simulink model "Task1_Simulink"  (R2023b)
settings: Solver=VariableStepAuto  StartTime=0.0  StopTime=10.0  RelTol=1e-3
values from neighbouring files (symbols this model uses):
  k = find(modeldata.studentList == studentNo)    [runExam.m]
undefined symbols (not defined in the file or in its folder): b, g, m, theta1, theta2, zk
settings Model: Creator=qnmdgpqs  LastModifiedBy=qnmdgpqs

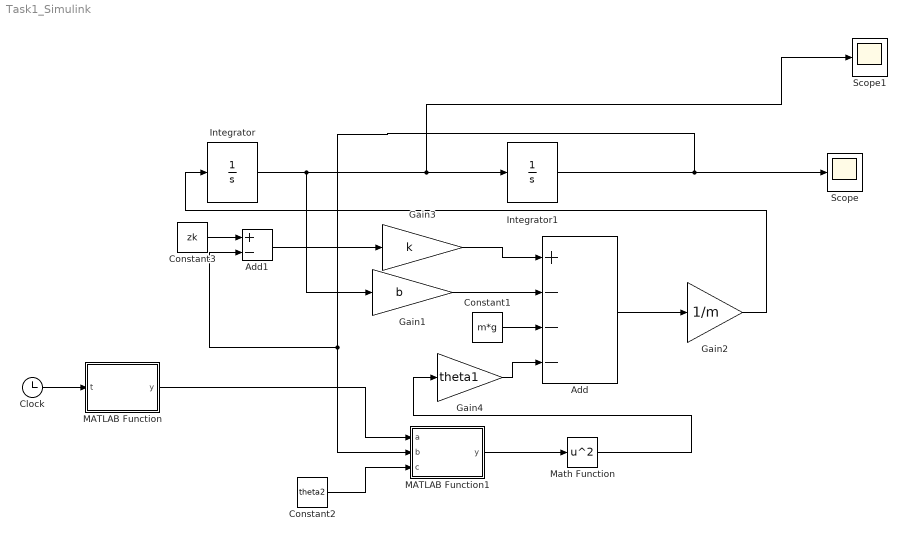
== system Task1_Simulink ==
  Add : Sum  Inputs=+---
  Add1 : Sum  Inputs=+-
  Clock : Clock
  Constant1 : Constant  Value=m*g
  Constant2 : Constant  Value=theta2
  Constant3 : Constant  Value=zk
  Gain1 : Gain  Gain=b
  Gain2 : Gain  Gain=1/m
  Gain3 : Gain  Gain=k
  Gain4 : Gain  Gain=theta1
  Integrator : Integrator
  Integrator1 : Integrator  InitialCondition=0.1
  MATLAB Function : MATLAB Function  TreatAsAtomicUnit=on
  MATLAB Function1 : MATLAB Function  TreatAsAtomicUnit=on
  Math Function : Math  Operator=square
  Scope : Scope
  Scope1 : Scope
  wires:
  Integrator1/1 -> MATLAB Function1/2(b), Add1/2, Scope/1
  Integrator/1 -> Scope1/1, Integrator1/1, Gain1/1
  Math Function/1 -> Gain4/1
  Gain1/1 -> Add/2
  Constant1/1 -> Add/3
  Gain4/1 -> Add/4
  Add/1 -> Gain2/1
  Gain2/1 -> Integrator/1
  Constant2/1 -> MATLAB Function1/3(c)
  Clock/1 -> MATLAB Function/1(t)
  Constant3/1 -> Add1/1
  Add1/1 -> Gain3/1
  Gain3/1 -> Add/1
  MATLAB Function/1(y) -> MATLAB Function1/1(a)
  MATLAB Function1/1(y) -> Math Function/1

== matlab function Task1_Simulink/MATLAB Function ==
  data: t input; y output
function y = fcn(t)

y = 10 * sin(10 * t);

== matlab function Task1_Simulink/MATLAB Function1 ==
  data: a input; y output; b input; c input
function y = fcn(a,b,c)

y = a/(b+c);
